simulink model "chap3_5sim"  (Simulink 3.00)
settings: Solver=FixedStepDiscrete  StartTime=0.0  StopTime=2  RelTol=1e-3
values from neighbouring files (symbols this model uses):
  A = [1 0.0010 ... (first row only)    [chap3_1.m]
  B = [-0.0001 ... (first row only)    [chap3_1.m]
  C = [c 1]    [chap3_1.m]
undefined symbols (not defined in the file or in its folder): D, T
settings Model: SaveTime=off  SaveOutput=off  Decimation=100  LastModifiedBy=liu

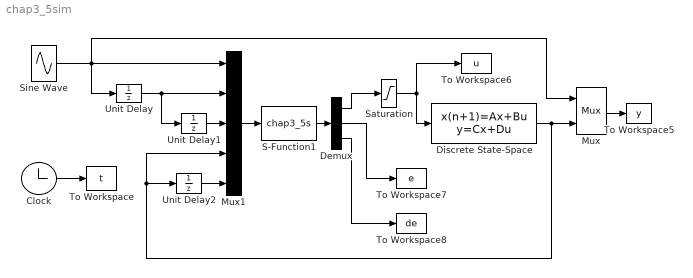
== system chap3_5sim ==
  Clock : Clock
  Demux : Demux  Outputs=3
  Discrete State-Space : DiscreteStateSpace  A=A  B=B  C=C  D=D  X0=[-0.5,-0.5]  SampleTime=T
  Mux : Mux  Inputs=2
      settings: DisplayOption=none
  Mux1 : Mux  Inputs=5
  S-Function1 : S-Function  FunctionName=chap3_5s  PortCounts=[]  SFunctionModules=''
  Saturation : Saturate  UpperLimit=10  LowerLimit=-10
  Sine Wave : Sin  Amplitude=0.5  Frequency=3*2*pi  Phase=0  SampleTime=0.001
  To Workspace : ToWorkspace  VariableName=t  SampleTime=-1  SaveFormat=Matrix
  To Workspace5 : ToWorkspace  VariableName=y  SampleTime=-1  SaveFormat=Matrix
  To Workspace6 : ToWorkspace  VariableName=u  SampleTime=-1  SaveFormat=Matrix
  To Workspace7 : ToWorkspace  VariableName=e  SampleTime=-1  SaveFormat=Matrix
  To Workspace8 : ToWorkspace  VariableName=de  SampleTime=-1  SaveFormat=Matrix
  Unit Delay : UnitDelay  X0=0  SampleTime=0.001
  Unit Delay1 : UnitDelay  X0=0  SampleTime=0.001
  Unit Delay2 : UnitDelay  X0=0  SampleTime=0.001
  wires:
  Mux/1 -> To Workspace5/1
  Mux1/1 -> S-Function1/1
  Discrete State-Space/1 -> Mux/2, Mux1/4, Unit Delay2/1
  Sine Wave/1 -> Mux/1, Unit Delay/1, Mux1/1
  Unit Delay1/1 -> Mux1/3
  Unit Delay/1 -> Mux1/2, Unit Delay1/1
  Unit Delay2/1 -> Mux1/5
  Clock/1 -> To Workspace/1
  S-Function1/1 -> Demux/1
  Demux/2 -> To Workspace7/1
  Demux/3 -> To Workspace8/1
  Demux/1 -> Saturation/1
  Saturation/1 -> Discrete State-Space/1, To Workspace6/1
